simulink model "observation1_simulink"  (R2020b)
settings: Solver=VariableStepAuto  StartTime=0.0  StopTime=0  RelTol=1e-3
settings Model: Creator=Mohit Akhouri  LastModifiedBy=Mohit Akhouri

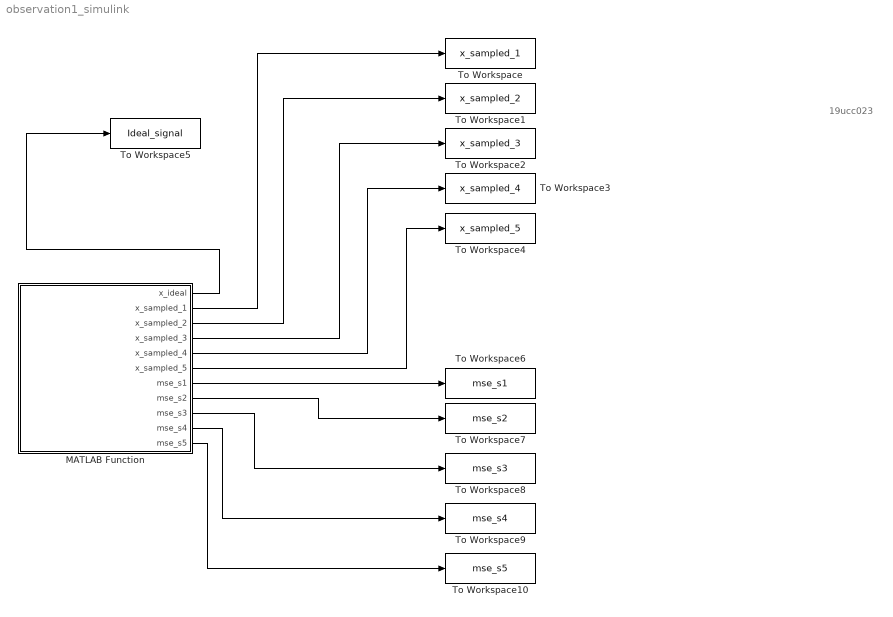
== system observation1_simulink ==
  note: 19ucc023
  MATLAB Function : MATLAB Function  TreatAsAtomicUnit=on
  To Workspace : ToWorkspace  VariableName=x_sampled_1  SaveFormat=Timeseries  SampleTime=-1
  To Workspace1 : ToWorkspace  VariableName=x_sampled_2  SaveFormat=Timeseries  SampleTime=-1
  To Workspace10 : ToWorkspace  VariableName=mse_s5  SaveFormat=Timeseries  SampleTime=-1
  To Workspace2 : ToWorkspace  VariableName=x_sampled_3  SaveFormat=Timeseries  SampleTime=-1
  To Workspace3 : ToWorkspace  VariableName=x_sampled_4  SaveFormat=Timeseries  SampleTime=-1
  To Workspace4 : ToWorkspace  VariableName=x_sampled_5  SaveFormat=Timeseries  SampleTime=-1
  To Workspace5 : ToWorkspace  VariableName=Ideal_signal  SaveFormat=Timeseries  SampleTime=-1
  To Workspace6 : ToWorkspace  VariableName=mse_s1  SaveFormat=Timeseries  SampleTime=-1
  To Workspace7 : ToWorkspace  VariableName=mse_s2  SaveFormat=Timeseries  SampleTime=-1
  To Workspace8 : ToWorkspace  VariableName=mse_s3  SaveFormat=Timeseries  SampleTime=-1
  To Workspace9 : ToWorkspace  VariableName=mse_s4  SaveFormat=Timeseries  SampleTime=-1
  wires:
  MATLAB Function/2(x_sampled_1) -> To Workspace/1
  MATLAB Function/3(x_sampled_2) -> To Workspace1/1
  MATLAB Function/4(x_sampled_3) -> To Workspace2/1
  MATLAB Function/5(x_sampled_4) -> To Workspace3/1
  MATLAB Function/6(x_sampled_5) -> To Workspace4/1
  MATLAB Function/1(x_ideal) -> To Workspace5/1
  MATLAB Function/7(mse_s1) -> To Workspace6/1
  MATLAB Function/8(mse_s2) -> To Workspace7/1
  MATLAB Function/9(mse_s3) -> To Workspace8/1
  MATLAB Function/10(mse_s4) -> To Workspace9/1
  MATLAB Function/11(mse_s5) -> To Workspace10/1

== matlab function observation1_simulink/MATLAB Function ==
  data: x_ideal output; x_sampled_1 output; x_sampled_2 output; x_sampled_3 output; x_sampled_4 output; x_sampled_5 output; mse_s1 output; mse_s2 output; mse_s3 output; mse_s4 output; mse_s5 output
function [x_ideal,x_sampled_1,x_sampled_2,x_sampled_3,x_sampled_4,x_sampled_5,mse_s1,mse_s2,mse_s3,mse_s4,mse_s5] = fcn()

A = 1; % defining amplitude
n_cycles = 5; % defining number of cycles
fs_ideal = 100000; % defining ideal frequency
f = 3000; % defining message signal frequency

% generating ideal signal

n_ideal = 0:1:floor(n_cycles*(fs_ideal/f))-1;
x_ideal = A*cos(2*pi*f*n_ideal*(1/fs_ideal));

% generating sampled signals
fs1 = 10000;
ns1 = 0:1:floor(n_cycles*(fs1/f))-1;
x_sampled_1 = A*cos(2*pi*f*ns1*(1/fs1)); % sampled signal 1

fs2 = 6000;
ns2 = 0:1:floor(n_cycles*(fs2/f))-1;
x_sampled_2 = A*cos(2*pi*f*ns2*(1/fs2)); % sampled signal 2

fs3 = 12000;
ns3 = 0:1:floor(n_cycles*(fs3/f))-1;
x_sampled_3 = A*cos(2*pi*f*ns3*(1/fs3)); % sampled signal 3

fs4 = 4000;
ns4 = 0:1:floor(n_cycles*(fs4/f))-1;
x_sampled_4 = A*cos(2*pi*f*ns4*(1/fs4)); % sampled signal 4

fs5 = 5000;
ns5 = 0:1:floor(n_cycles*(fs5/f))-1;
x_sampled_5 = A*cos(2*pi*f*ns5*(1/fs5)); % sampled signal 5

% generating the parameters x and xq for use in interp1 function for
% different sampling rates
x_s1 = 0:1:max(ns1);
xq_s1 = 0:max(ns1)/max(n_ideal):max(ns1);

x_s2 = 0:1:max(ns2);
xq_s2 = 0:max(ns2)/max(n_ideal):max(ns2);

x_s3 = 0:1:max(ns3);
xq_s3 = 0:max(ns3)/max(n_ideal):max(ns3);

x_s4 = 0:1:max(ns4);
xq_s4 = 0:max(ns4)/max(n_ideal):max(ns4);

x_s5 = 0:1:max(ns5);
xq_s5 = 0:max(ns5)/max(n_ideal):max(ns5);

inter_method = 'linear'; % using linear interpolation method

inter_s1 = interp1(x_s1,x_sampled_1,xq_s1,inter_method); % interpolated signal for Fs = 10000 Hz
inter_s2 = interp1(x_s2,x_sampled_2,xq_s2,inter_method); % interpolated signal for Fs = 6000 Hz
inter_s3 = interp1(x_s3,x_sampled_3,xq_s3,inter_method); % interpolated signal for Fs = 12000 Hz
inter_s4 = interp1(x_s4,x_sampled_4,xq_s4,inter_method); % interpolated signal for Fs = 4000 Hz
inter_s5 = interp1(x_s5,x_sampled_5,xq_s5,inter_method); % interpolated signal for Fs = 5000 Hz

mse_s1 = mean((x_ideal - inter_s1).^2); % MSE for Fs = 10000 Hz
mse_s2 = mean((x_ideal - inter_s2).^2); % MSE for Fs = 6000 Hz
mse_s3 = mean((x_ideal - inter_s3).^2); % MSE for Fs = 12000 Hz
mse_s4 = mean((x_ideal - inter_s4).^2); % MSE for Fs = 4000 Hz
mse_s5 = mean((x_ideal - inter_s5).^2); % MSE for Fs = 5000 Hz
